simulink model "airbrake_sim"  (R2024b)
settings: Solver=FixedStepAuto  StartTime=0.0  StopTime=8  FixedStep=0.001  RelTol=1e-3
model workspace (MAT data in the model file):
  shutoff_time = 2
settings Model: Creator=joshuabeard  LastModifiedBy=joshuabeard

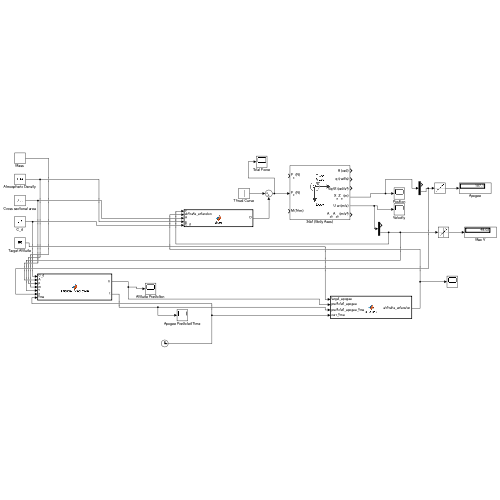
[thumbnail: Simulink's stored preview of the top-level diagram]
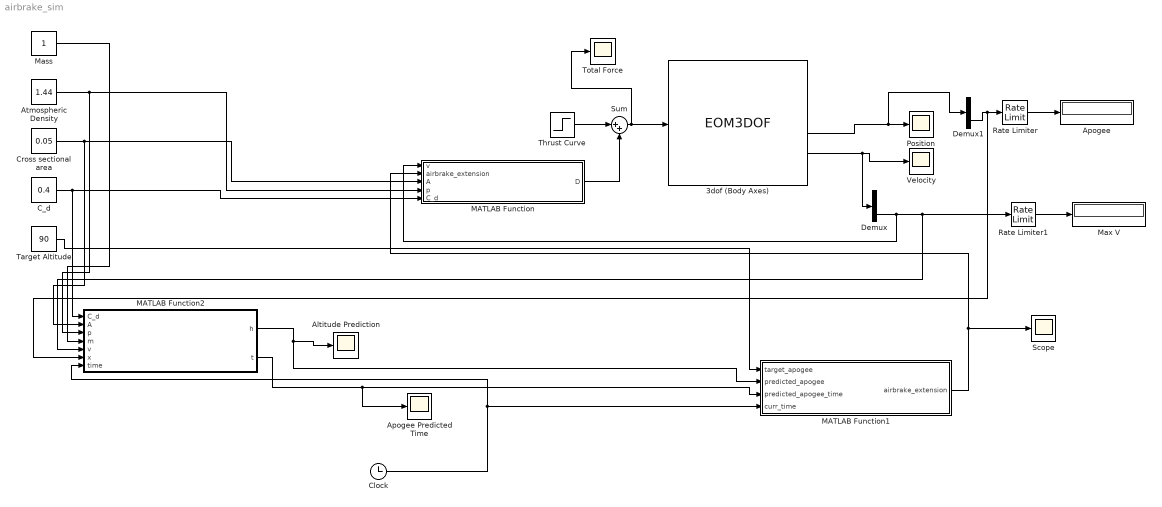
== system airbrake_sim ==
  3dof (Body Axes) : EOM3DOF  v_ini=0  g=-9.81
  Altitude Prediction : Scope
  Apogee : Display
  Apogee Predicted Time : Scope
  Atmospheric Density : Constant  Value=1.44
  C_d : Constant  Value=0.4
  Clock : Clock
  Cross sectional area : Constant  Value=0.05
  Demux : Demux  Outputs=2
  Demux1 : Demux  Outputs=2
  MATLAB Function : MATLAB Function  TreatAsAtomicUnit=on
  MATLAB Function1 : MATLAB Function  TreatAsAtomicUnit=on
  MATLAB Function2 : MATLAB Function  TreatAsAtomicUnit=on
  Mass : Constant
  Max V : Display
  Position : Scope
  Rate Limiter : RateLimiter  RisingSlewLimit=99999  FallingSlewLimit=0  SampleTimeMode=inherited
  Rate Limiter1 : RateLimiter  RisingSlewLimit=999999  FallingSlewLimit=0  SampleTimeMode=inherited
  Scope : Scope
  Sum : Sum  Inputs=|++
  Target Altitude : Constant  Value=90
  Thrust Curve : Step  Time=2  Before=50  After=0  SampleTime=0
  Total Force : Scope
  Velocity : Scope
  wires:
  3dof (Body Axes)/4 -> Demux1/1, Position/1
  3dof (Body Axes)/5 -> Demux/1, Velocity/1
  Thrust Curve/1 -> Sum/1
  Sum/1 -> Total Force/1, 3dof (Body Axes)/2
  MATLAB Function/1(D) -> Sum/2
  Demux/2 -> MATLAB Function2/5(v), Rate Limiter1/1, MATLAB Function/1(v)
  Demux1/2 -> MATLAB Function2/6(x), Rate Limiter/1
  Rate Limiter/1 -> Apogee/1
  MATLAB Function1/1(airbrake_extension) -> Scope/1, MATLAB Function/2(airbrake_extension)
  Rate Limiter1/1 -> Max V/1
  Target Altitude/1 -> MATLAB Function1/1(target_apogee)
  Cross sectional area/1 -> MATLAB Function2/2(A), MATLAB Function/3(A)
  C_d/1 -> MATLAB Function2/1(C_d), MATLAB Function/5(C_d)
  Atmospheric Density/1 -> MATLAB Function2/3(p), MATLAB Function/4(p)
  Mass/1 -> MATLAB Function2/4(m)
  MATLAB Function2/1(h) -> MATLAB Function1/2(predicted_apogee), Altitude Prediction/1
  Clock/1 -> MATLAB Function2/7(time), MATLAB Function1/4(curr_time)
  MATLAB Function2/2(t) -> Apogee Predicted Time/1, MATLAB Function1/3(predicted_apogee_time)

== matlab function airbrake_sim/MATLAB Function1 ==
  data: airbrake_extension output; target_apogee input; predicted_apogee input; predicted_apogee_time input; curr_time input
function airbrake_extension  = airbrake(target_apogee, predicted_apogee, predicted_apogee_time, curr_time)
P = 1;
I = 0;
D = 0;

airbrake_extension = 0;

if (curr_time > 2) && (curr_time < predicted_apogee_time)


    error = predicted_apogee - target_apogee;
    airbrake_extension = min(max((P * error),0),1);

end

airbrake_extension = 0;
end

== matlab function airbrake_sim/MATLAB Function ==
  data: v input; D output; airbrake_extension input; A input; p input; C_d input
function D = drag(v, airbrake_extension, A, p, C_d)


Cd = C_d + airbrake_extension * 0.9; % or whatever function interpolates between closed and open airbrakes

D = -1 * (1/2) * Cd * p * A * (v^2);

end

== matlab function airbrake_sim/MATLAB Function2 ==
  data: C_d input; h output; A input; p input; m input; v input; x input; t output; time input
function [h, t] = altitude_prediction(C_d, A, p, m, v, x, time)
% predicts altitude given current position and velocity.  Accounts for drag
k = (1/2) * (C_d * A * p) / m;
a = 9.81;
c_1 = (atan(sqrt(k/a) * v * -1))/(sqrt(a * k)); % -1 * time until apogee
c_2 = x - (1/k) * (log(cos(c_1 * sqrt(a * k)))); % height of apogee

t = -1 * c_1 + time;
h = c_2;
end
